simulink subsystem "DAC"  (R2023a)
settings: Solver=VariableStepAuto  StartTime=0.0  StopTime=10.0  RelTol=1e-3
libraries: dspsigops x1
settings Model: Creator=diontep  LastModifiedBy=diontep

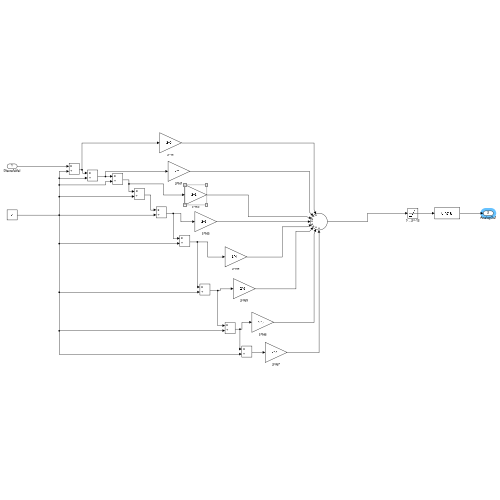
[thumbnail: Simulink's stored preview of the top-level diagram]
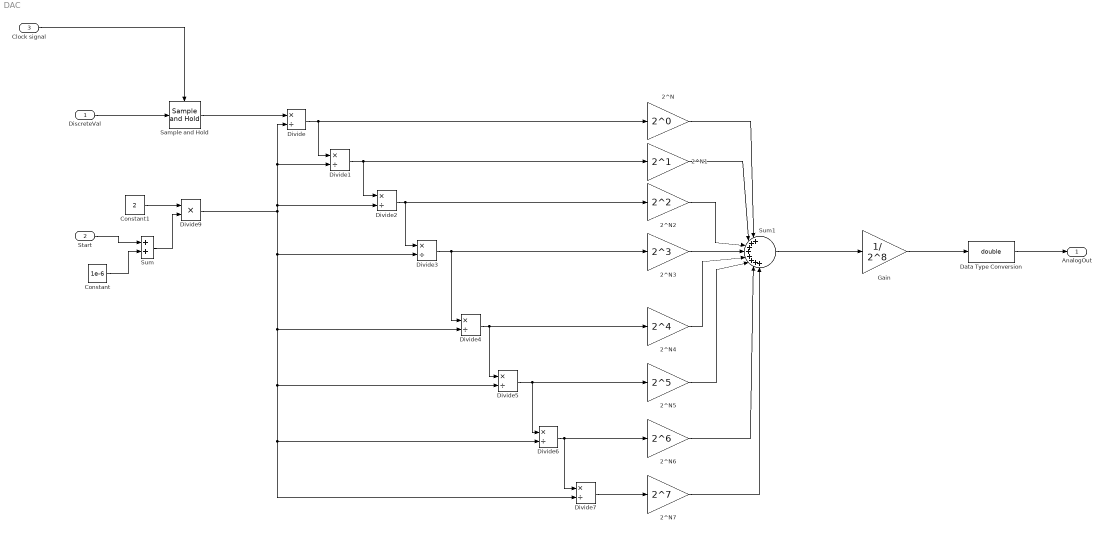
== system DAC ==
  DiscreteVal : Inport
  Start : Inport  Port=2
  Clock signal : Inport  Port=3
  2^N : Gain  Gain=2^0
  2^N1 : Gain  Gain=2^1
  2^N2 : Gain  Gain=2^2
  2^N3 : Gain  Gain=2^3
  2^N4 : Gain  Gain=2^4
  2^N5 : Gain  Gain=2^5
  2^N6 : Gain  Gain=2^6
  2^N7 : Gain  Gain=2^7
  Constant : Constant  Value=1e-6
  Constant1 : Constant  Value=2
  Data Type Conversion : DataTypeConversion  OutDataTypeStr=double  SaturateOnIntegerOverflow=off  RndMeth=Floor
  Divide{,1..7} (8 alike) : Product  Inputs=*/
  Divide9 : Product  Inputs=**
  Gain : Gain  Gain=1/ 2^8
  Sample and Hold : dspsigops/Sample and Hold  trig=Rising edge  initCond=0  latchinput=off
  Sum : Sum
  Sum1 : Sum  Inputs=|++++++++
  AnalogOut : Outport
  wires:
  2^N5/1 -> Sum1/6
  Divide/1 -> Divide1/1, 2^N/1
  2^N3/1 -> Sum1/4
  Divide3/1 -> Divide4/1, 2^N3/1
  Divide6/1 -> Divide7/1, 2^N6/1
  2^N2/1 -> Sum1/3
  Divide5/1 -> Divide6/1, 2^N5/1
  Divide1/1 -> Divide2/1, 2^N1/1
  2^N7/1 -> Sum1/8
  Sum1/1 -> Gain/1
  Divide2/1 -> Divide3/1, 2^N2/1
  Divide4/1 -> Divide5/1, 2^N4/1
  2^N/1 -> Sum1/1
  2^N1/1 -> Sum1/2
  Divide9/1 -> Divide2/2, Divide1/2, Divide/2, Divide4/2, Divide5/2, Divide6/2, Divide7/2, Divide3/2
  2^N4/1 -> Sum1/5
  2^N6/1 -> Sum1/7
  Divide7/1 -> 2^N7/1
  Constant/1 -> Sum/2
  Sum/1 -> Divide9/2
  Start/1 -> Sum/1
  Constant1/1 -> Divide9/1
  Data Type Conversion/1 -> AnalogOut/1
  Gain/1 -> Data Type Conversion/1
  Clock signal/1 -> Sample and Hold/Trigger
  Sample and Hold/1 -> Divide/1
  DiscreteVal/1 -> Sample and Hold/1
